simulink model "version1_dischargeckt"  (R2021b)
settings: Solver=VariableStepAuto  StartTime=0.0  StopTime=7000  RelTol=1e-3
undefined symbols (not defined in the file): Ion, Lithium
libraries: spsBatteryLib x3, spsCurrentMeasurementLib x1, spsMosfetLib x1, spsSeriesRLCBranchLib x1, spsVoltageMeasurementLib x1, spspowerguiLib x1
settings Model: Creator=Aashish Kalra  LastModifiedBy=Admin
settings SolverCC: AlgebraicLoopSolver=TrustRegion
settings DataIOCC: ReturnWorkspaceOutputs=off
settings DebuggingCC: SFMachineParentedDataDiag=warning  ArithmeticOperatorsInVariantConditions=warning
settings SFSimCC: SimUseLocalCustomCode=off  CustomCodeUndefinedFunction=UseInterfaceOnly
settings RTWCC: RTWUseLocalCustomCode=off

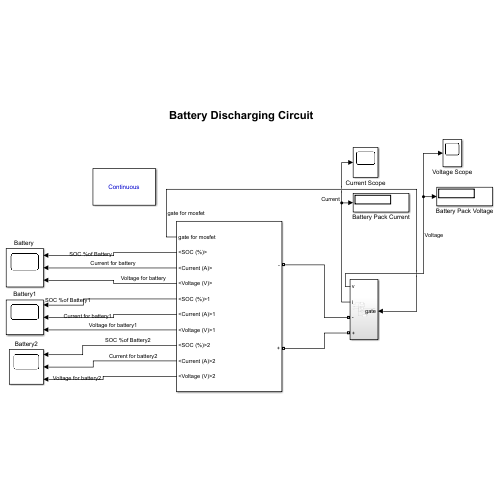
[thumbnail: Simulink's stored preview of the top-level diagram]
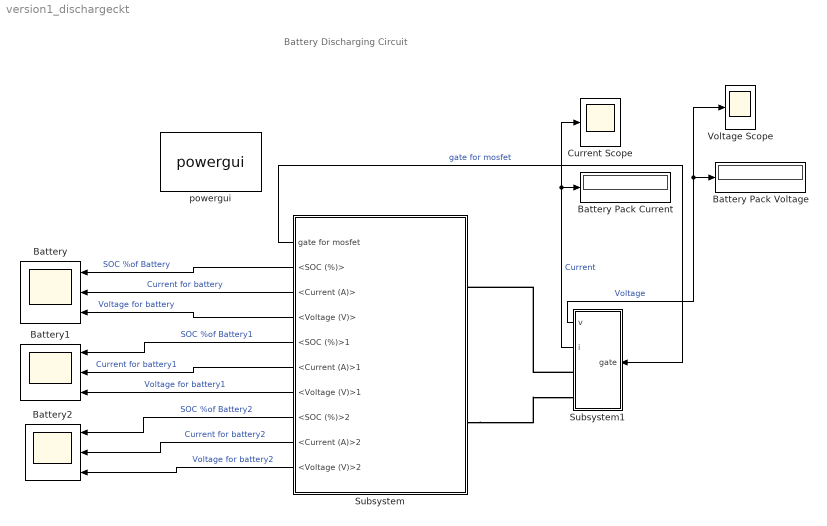
== system version1_dischargeckt ==
  note: Battery Discharging Circuit
  "Battery " : Scope  NumInputPorts=3
  Battery Pack Current : Display
  Battery Pack Voltage : Display
  Battery1 : Scope  NumInputPorts=3
  Battery2 : Scope  NumInputPorts=3
  Current Scope : Scope
  Subsystem : Subsystem
  Subsystem1 : Subsystem
  Voltage Scope : Scope
  powergui : spspowerguiLib/powergui  Priority=1  SimulationMode=Continuous  SampleTime=50e-6  frequency=60  Iterations=50  frequencyindice=0  Pbase=100e6  ErrMax=1e-4  UnitsV=kV  UnitsW=MW  buscounter=0  FunctionMessages=off  echomessages=off  EnableUseOfTLC=off  CurrentSourceSwitches=off  DisableSnubberDevices=off  DisableRonSwitches=off  DisableVfSwitches=off  DisplayEquations=off  AutomaticDiscreteSolvers=off  SolverType=Tustin/Backward Euler (TBE)  Interpol=off  ExternalGateDelay=off  methode=off  Ts=100  x0status=blocks  SPID=on  SwTol=0  HookPort=off  NonlinearTolerance=1e-4  nMaxIteration=100  ContinueOnMaxIteration=off  RestoreLinks=warning  ResistiveCurrentMeasurement=off  Frange=[0:2:500]  Ylog=off  Xlog=on  ShowGrid=off  save=off  variable=ZData  structure=0  ZoomFFT=off  StartTime=0.0  cycles=1  DisplayStyle=1  fundamental=60  FreqAxis=off  MaxFrequency=1000  frequencyindicesteady=1  RmsSteady=1  display=off
  wires:
  Subsystem/2(<SOC (%)>) -> "Battery "/1  "SOC %of Battery"
  Subsystem/3(<Current (A)>) -> "Battery "/2  "Current for battery"
  Subsystem/4(<Voltage (V)>) -> "Battery "/3  "Voltage for battery"
  Subsystem/5(<SOC (%)>1) -> Battery1/1  "SOC %of Battery1"
  Subsystem/6(<Current (A)>1) -> Battery1/2  "Current for battery1"
  Subsystem/7(<Voltage (V)>1) -> Battery1/3  "Voltage for battery1"
  Subsystem/8(<SOC (%)>2) -> Battery2/1  "SOC %of Battery2"
  Subsystem/9(<Current (A)>2) -> Battery2/2  "Current for battery2"
  Subsystem/10(<Voltage (V)>2) -> Battery2/3  "Voltage for battery2"
  Subsystem1/1(v) -> Battery Pack Voltage/1, Voltage Scope/1  "Voltage"
  Subsystem1/2(i) -> Current Scope/1, Battery Pack Current/1  "Current"
  Subsystem/1(gate for mosfet) -> Subsystem1/1(gate)  "gate for mosfet"
  connections:
  Subsystem1/RConn1 -- Subsystem/LConn1
  Subsystem/LConn2 -- Subsystem1/RConn2

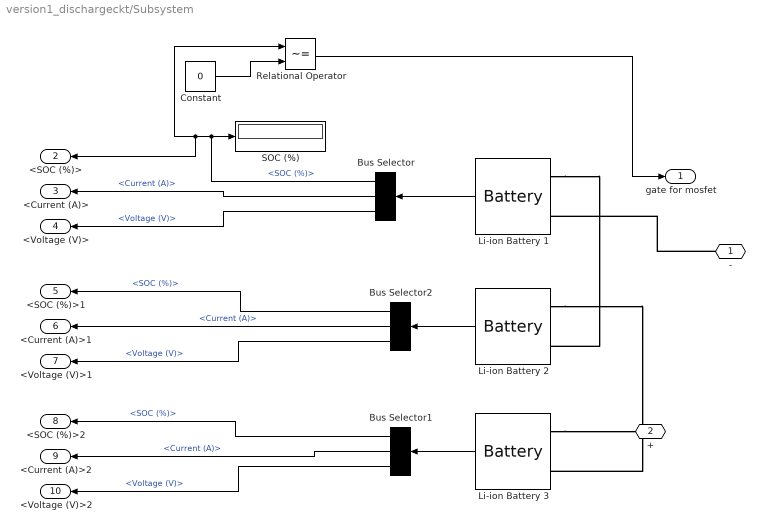
== system version1_dischargeckt/Subsystem ==
  Bus Selector : BusSelector  OutputSignals=SOC (%),Current (A),Voltage (V)
  Bus Selector1 : BusSelector  OutputSignals=SOC (%),Current (A),Voltage (V)
  Bus Selector2 : BusSelector  OutputSignals=SOC (%),Current (A),Voltage (V)
  Constant : Constant  Value=0
  Li-ion Battery 1 : spsBatteryLib/Battery  BatType=Lithium-Ion  ShowTempParam=off  ThermalPreset=no  ShowAgeParam=off  NomV=3.7  NomQ=2.6  SOC=96  Batt_Tr=30  PresetModel=on  MaxQ=2.6  MinV=2.775  FullV=4.3068  Dis_rate=1.1304  R=0.014231  Normal_OP=2.3513  expZone="[3.9974     0.12774]"  current=[6.5 13 32.5]  Units=Time  Tci=20  NomT=20  T2=-30  MaxQ2=4.8  FullV2=7.1  Normal_OP2=5.655  expZone2="[6.58           1]"  Rca=0.6  ti=2000  Dp=0  Neq0=0  Tsim=1e6  Ta1=25  Qeol=5.4*0.9  Reol=0.013333*1.2  Char_age=[2.3478, 3]  Dis_age=[2.3478, 10]  N1=1500  N2=10500  N3=1000  N4=1400  Ta2=45  N5=950
  Li-ion Battery 2 : spsBatteryLib/Battery  BatType=Lithium-Ion  ShowTempParam=off  ThermalPreset=no  ShowAgeParam=off  NomV=3.7  NomQ=2.6  SOC=96  Batt_Tr=30  PresetModel=on  MaxQ=2.6  MinV=2.775  FullV=4.3068  Dis_rate=1.1304  R=0.014231  Normal_OP=2.3513  expZone="[3.9974     0.12774]"  current=[6.5 13 32.5]  Units=Time  Tci=20  NomT=20  T2=-30  MaxQ2=4.8  FullV2=7.1  Normal_OP2=5.655  expZone2="[6.58           1]"  Rca=0.6  ti=2000  Dp=0  Neq0=0  Tsim=1e6  Ta1=25  Qeol=5.4*0.9  Reol=0.013333*1.2  Char_age=[2.3478, 3]  Dis_age=[2.3478, 10]  N1=1500  N2=10500  N3=1000  N4=1400  Ta2=45  N5=950
  Li-ion Battery 3 : spsBatteryLib/Battery  BatType=Lithium-Ion  ShowTempParam=off  ThermalPreset=no  ShowAgeParam=off  NomV=3.7  NomQ=2.6  SOC=96  Batt_Tr=30  PresetModel=on  MaxQ=2.6  MinV=2.775  FullV=4.3068  Dis_rate=1.1304  R=0.014231  Normal_OP=2.3513  expZone="[3.9974     0.12774]"  current=[6.5 13 32.5]  Units=Time  Tci=20  NomT=20  T2=-30  MaxQ2=4.8  FullV2=7.1  Normal_OP2=5.655  expZone2="[6.58           1]"  Rca=0.6  ti=2000  Dp=0  Neq0=0  Tsim=1e6  Ta1=25  Qeol=5.4*0.9  Reol=0.013333*1.2  Char_age=[2.3478, 3]  Dis_age=[2.3478, 10]  N1=1500  N2=10500  N3=1000  N4=1400  Ta2=45  N5=950
  Relational Operator : RelationalOperator  Operator=~=  OutDataTypeStr=boolean  RndMeth=Simplest
  SOC (%) : Display
  - : PMIOPort  Side=Left
  + : PMIOPort  Port=2  Side=Left
  gate for mosfet : Outport
  <SOC (%)> : Outport  Port=2
  <Current (A)> : Outport  Port=3
  <Voltage (V)> : Outport  Port=4
  <SOC (%)>1 : Outport  Port=5
  <Current (A)>1 : Outport  Port=6
  <Voltage (V)>1 : Outport  Port=7
  <SOC (%)>2 : Outport  Port=8
  <Current (A)>2 : Outport  Port=9
  <Voltage (V)>2 : Outport  Port=10
  wires:
  Li-ion Battery 2/1 -> Bus Selector2/1
  Li-ion Battery 3/1 -> Bus Selector1/1
  Relational Operator/1 -> gate for mosfet/1
  Bus Selector/1 -> <SOC (%)>/1, Relational Operator/1, SOC (%)/1  "<SOC (%)>"
  Li-ion Battery 1/1 -> Bus Selector/1
  Constant/1 -> Relational Operator/2
  Bus Selector/3 -> <Voltage (V)>/1  "<Voltage (V)>"
  Bus Selector2/3 -> <Voltage (V)>1/1  "<Voltage (V)>"
  Bus Selector1/1 -> <SOC (%)>2/1  "<SOC (%)>"
  Bus Selector/2 -> <Current (A)>/1  "<Current (A)>"
  Bus Selector1/2 -> <Current (A)>2/1  "<Current (A)>"
  Bus Selector2/1 -> <SOC (%)>1/1  "<SOC (%)>"
  Bus Selector1/3 -> <Voltage (V)>2/1  "<Voltage (V)>"
  Bus Selector2/2 -> <Current (A)>1/1  "<Current (A)>"
  connections:
  Li-ion Battery 2/LConn1 -- Li-ion Battery 3/LConn2
  Li-ion Battery 1/LConn1 -- Li-ion Battery 2/LConn2
  Li-ion Battery 3/LConn1 -- +/RConn1
  -/RConn1 -- Li-ion Battery 1/LConn2

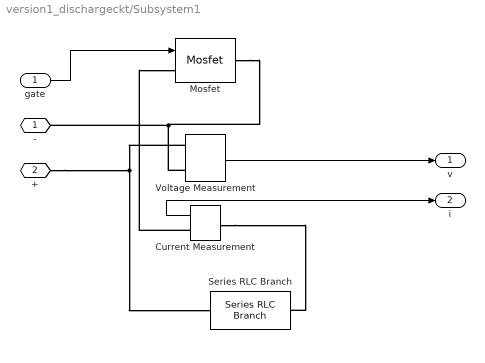
== system version1_dischargeckt/Subsystem1 ==
  gate : Inport
  Current Measurement : spsCurrentMeasurementLib/Current Measurement  PhasorSimulation=off  OutputType=Complex  PSBequivalent=0
  Mosfet : spsMosfetLib/Mosfet  Ron=0.1  Lon=0  Rd=0.01  Vfd=0  IC=0  Rs=1e5  Cs=inf  Measurements=off
  Series RLC Branch : spsSeriesRLCBranchLib/Series RLC Branch  LConnTagsString=__new0  RConnTagsString=__new0  BranchType=R  Resistance=4.6  Inductance=1e-3  SetiL0=off  InitialCurrent=0  Capacitance=1e-6  Setx0=off  InitialVoltage=0  Measurements=None
  Voltage Measurement : spsVoltageMeasurementLib/Voltage Measurement  PhasorSimulation=off  OutputType=Complex  PSBequivalent=0
  - : PMIOPort  Side=Right
  + : PMIOPort  Port=2  Side=Right
  v : Outport
  i : Outport  Port=2
  wires:
  Voltage Measurement/1 -> v/1
  gate/1 -> Mosfet/1
  Current Measurement/1 -> i/1
  connections:
  Voltage Measurement/LConn1 -- +/RConn1 -- Series RLC Branch/RConn1
  Mosfet/RConn1 -- Voltage Measurement/LConn2 -- -/RConn1
  Current Measurement/RConn1 -- Mosfet/LConn1
  Current Measurement/LConn1 -- Series RLC Branch/LConn1
